simulink model "work1"  (R2016b)
settings: Solver=FixedStepDiscrete  StartTime=0.0  StopTime=1024  FixedStep=0.0015625  RelTol=1e-3
libraries: dspmlti4 x2, dspsrcs4 x2, dspstat3 x1, dsparch4 x1
settings Model: Creator=AreVa  LastModifiedBy=AreVa
settings SolverCC: AutoInsertRateTranBlk=on
settings OptimizationCC: DefaultParameterBehavior=Inlined  InlineInvariantSignals=on  EfficientFloat2IntCast=on
settings ConfigComp: CovScope=ReferencedModels  CovIncludeTopModel=off

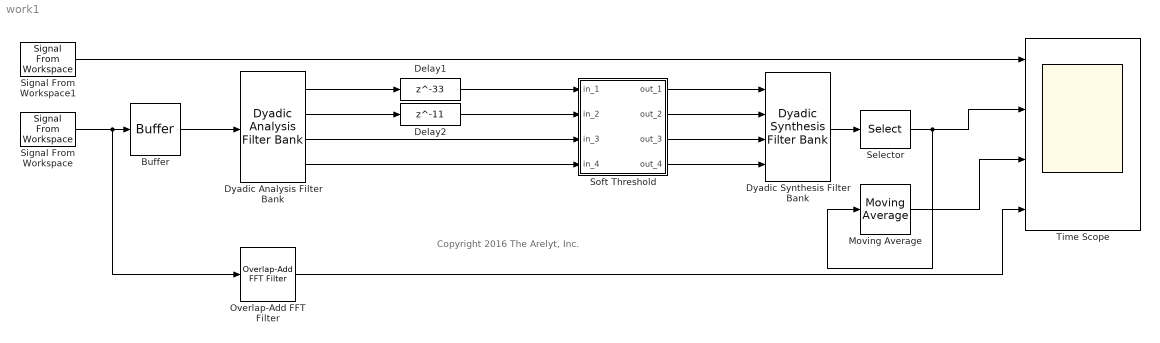
== system work1 ==
  note: Copyright 2016 The Arelyt, Inc.
  Buffer : Buffer  V=63  TreatMby1Signals=One channel  OutputFrames=off
  Delay1 : Delay  DelayLength=33  InitialCondition=0  InputProcessing=Columns as channels (frame based)
  Delay2 : Delay  DelayLength=11  InitialCondition=0  InputProcessing=Columns as channels (frame based)
  Dyadic Analysis Filter Bank : dspmlti4/Dyadic Analysis Filter Bank  Wname=Biorthogonal  OrdRec_ordDec=[3 / 5]  Order=2  LPF=lod  HPF=hid  NumLevels=3  tree=Asymmetric  Output=Multiple ports  OutputFrames=off
  Dyadic Synthesis Filter Bank : dspmlti4/Dyadic Synthesis Filter Bank  Wname=Biorthogonal  OrdRec_ordDec=[3 / 5]  Order=2  LPF=lor  HPF=hir  NumLevels=3  tree=Asymmetric  Input=Multiple ports  OutputFrames=off
  Moving Average : dspstat3/Moving Average  Method=Sliding window  SpecifyWindowLength=on  WindowLength=4  ForgettingFactor=0.9  SimulateUsing=Code generation
  Overlap-Add FFT Filter : dsparch4/Overlap-Add FFT Filter  Nfft=64  h=fir1(20,0.2)  output_complexity=Real  TreatMby1Signals=One channel
  Selector : Selector  InputPortWidth=64  IndexOptions=Index vector (dialog)  Indices=[1]  OutputSizes=1
  Signal From Workspace : dspsrcs4/Signal From Workspace  X=signal  Ts=1  nsamps=1  OutputAfterFinalValue=Holding final value  ignoreOrWarnInputAndFrameLengths=off  OutputFrames=off
  Signal From Workspace1 : dspsrcs4/Signal From Workspace  X=price  Ts=1  nsamps=1  OutputAfterFinalValue=Holding final value  ignoreOrWarnInputAndFrameLengths=off  OutputFrames=off
  Soft Threshold : Subsystem  mask(Soft Threshold){st=[3.694 2.803 1.411 0]}
      mask prompts: st "Vector of thresholds for each level:"
      mask help: Apply a soft threshold (deadzone transfer function) to each signal in the decomposition. First threshold applies to top-most filter bank output.
      mask init:
      | x=([-1 1 NaN 0 0 NaN -1 -.5 .5 1]+1)/2*.7+.15;
      | y=([0 0 NaN -1 1 NaN -1 0 0 1]+1)/2*.7+.05;
      mask Help: Vector of thresholds for each decomposition level.
      mask Display:
      | text(.1,.9,'Dead Zone')
      | plot(x,y)
  Time Scope : Scope  NumInputPorts=4
  wires:
  Signal From Workspace/1 -> Overlap-Add FFT Filter/1, Buffer/1
  Dyadic Analysis Filter Bank/1 -> Delay1/1
  Dyadic Analysis Filter Bank/2 -> Delay2/1
  Dyadic Analysis Filter Bank/4 -> Soft Threshold/4(in_4)
  Soft Threshold/4(out_4) -> Dyadic Synthesis Filter Bank/4
  Dyadic Analysis Filter Bank/3 -> Soft Threshold/3(in_3)
  Soft Threshold/3(out_3) -> Dyadic Synthesis Filter Bank/3
  Delay2/1 -> Soft Threshold/2(in_2)
  Soft Threshold/2(out_2) -> Dyadic Synthesis Filter Bank/2
  Delay1/1 -> Soft Threshold/1(in_1)
  Soft Threshold/1(out_1) -> Dyadic Synthesis Filter Bank/1
  Buffer/1 -> Dyadic Analysis Filter Bank/1
  Signal From Workspace1/1 -> Time Scope/1
  Dyadic Synthesis Filter Bank/1 -> Selector/1
  Selector/1 -> Moving Average/1, Time Scope/2
  Moving Average/1 -> Time Scope/3
  Overlap-Add FFT Filter/1 -> Time Scope/4

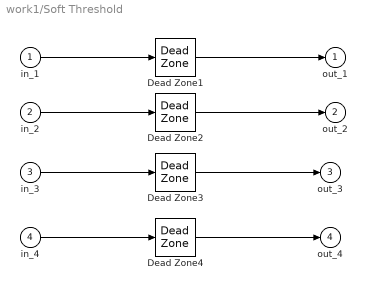
== system work1/Soft Threshold ==
  in_1 : Inport
  in_2 : Inport  Port=2
  in_3 : Inport  Port=3
  in_4 : Inport  Port=4
  Dead Zone1 : DeadZone  LowerValue=-st(1)  UpperValue=st(1)  ZeroCross=off  SaturateOnIntegerOverflow=on
  Dead Zone2 : DeadZone  LowerValue=-st(2)  UpperValue=st(2)  ZeroCross=off  SaturateOnIntegerOverflow=on
  Dead Zone3 : DeadZone  LowerValue=-st(3)  UpperValue=st(3)  ZeroCross=off  SaturateOnIntegerOverflow=on
  Dead Zone4 : DeadZone  LowerValue=-st(4)  UpperValue=st(4)  ZeroCross=off  SaturateOnIntegerOverflow=on
  out_1 : Outport
  out_2 : Outport  Port=2
  out_3 : Outport  Port=3
  out_4 : Outport  Port=4
  wires:
  in_1/1 -> Dead Zone1/1
  in_2/1 -> Dead Zone2/1
  in_3/1 -> Dead Zone3/1
  in_4/1 -> Dead Zone4/1
  Dead Zone1/1 -> out_1/1
  Dead Zone2/1 -> out_2/1
  Dead Zone3/1 -> out_3/1
  Dead Zone4/1 -> out_4/1
